simulink model "Model2"  (R2020a)
settings: Solver=VariableStepAuto  StartTime=0.0  StopTime=16*(1.302083333333333e-07)  RelTol=1e-3
undefined symbols (not defined in the file or in its folder): doppler, pskmod
libraries: commchan3 x2, commdigbbndpm3 x2, commutil2 x2, commrandsrc3 x1, commrflib2 x1, commsink2 x1
settings Model: Creator=esha_  LastModifiedBy=esha_

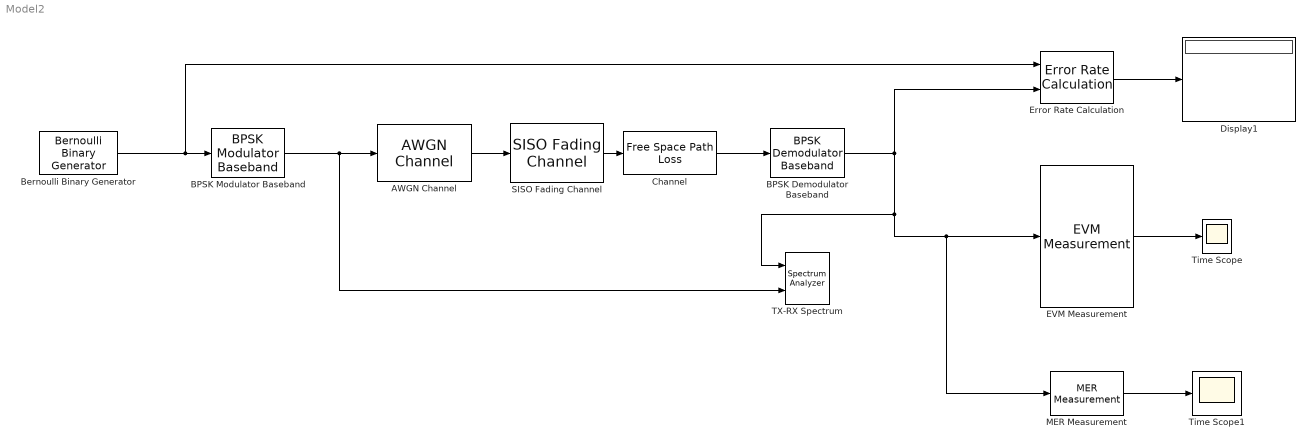
== system Model2 ==
  AWGN Channel : commchan3/AWGN Channel  InputProcessing=Columns as channels (frame based)  seed=67  noiseMode="Signal to noise ratio  (Eb/No)"  EbNodB=1  EsNodB=10  SNRdB=10  bitsPerSym=1  Ps=1  Tsym=0.000000065  variance=1
  BPSK Demodulator Baseband : commdigbbndpm3/BPSK Demodulator Baseband  DecType=Hard decision  VarSource=Dialog  Variance=1  Ph=0  outDtype=Inherit via internal rule  derotateFactorWordLen=16  derotateFactorDataTypeStr=Inherit: Same word length as input  derotateFactorLastDataTypeStr=Inherit: Same word length as input
  BPSK Modulator Baseband : commdigbbndpm3/BPSK Modulator Baseband  Ph=0  outDtype=double  outWordLen=16  outUDDataType=sfix(16)  outFracLenMode=Best precision  outFracLen=15  outDataTypeStr=double  outLastDataTypeStr=double
  Bernoulli Binary Generator : commrandsrc3/Bernoulli Binary Generator  ProbabilityOfZero=0.5  SeedSource=Parameter  Seed=61  SampleTime=1.302083333333333e-07  SamplesPerFrame=5000  OutputDataType=double  SimulateUsing=Code generation
  Channel : commrflib2/Free Space Path Loss  mode=Decibels  dB=50  d=0.100  fc=1920
      settings: SourceProductBaseCode=CM
  Display1 : Display
  EVM Measurement : commutil2/EVM Measurement  Normalization=Average reference signal power  AverageConstellationPower=1  PeakConstellationPower=1  ReferenceSignalSource=Estimated from reference constellation  ReferenceConstellation=pskmod((0:1),2,0)  MeasurementIntervalSource=Input length  MeasurementInterval=100  AveragingDimensions=1  MaximumEVMOutputPort=off  XPercentileEVMOutputPort=off  XPercentileValue=95  SymbolCountOutputPort=on  SimulateUsing=Interpreted execution
      settings: SourceProductBaseCode=CM
  Error Rate Calculation : commsink2/Error Rate Calculation  N=0  st_delay=0  cp_mode=Entire frame  subframe=[]  PMode=Port  WsName=ErrorVec  RsMode2=off  stop=on  numErr=100  maxBits=1e6
  MER Measurement : commutil2/MER Measurement  ReferenceSignalSource=Estimated from reference constellation  ReferenceConstellation=pskmod((0:1),2,0)  MeasurementIntervalSource=Input length  MeasurementInterval=100  AveragingDimensions=1  MinimumMEROutputPort=off  XPercentileMEROutputPort=off  XPercentileValue=95  SymbolCountOutputPort=off  SimulateUsing=Interpreted execution
      settings: SourceProductBaseCode=CM
  SISO Fading Channel : commchan3/SISO Fading Channel  InheritSampleRate=on  SampleRate=1  PathDelays=1.0e-06 *[0 0.2 0.4 0.8]  AveragePathGains="[0    -3    -6    -9]"  NormalizePathGains=on  FadingDistribution=Rayleigh  KFactor=3  DirectPathDopplerShift=0  DirectPathInitialPhase=0  MaximumDopplerShift=0.001  DopplerSpectrum=doppler('Jakes')  RandomStream=mt19937ar with seed  Seed=61  PathGainsOutputPort=off  ChannelFilterDelayOutputPort=off  SimulateUsing=Interpreted execution  Visualization=Frequency response  PathsForDopplerDisplay=1  SamplesToDisplay=100%
  TX-RX Spectrum : SpectrumAnalyzer  NumInputPorts=2
  Time Scope : Scope
      settings: Description=EVM
  Time Scope1 : Scope
      settings: Description=SNR
  wires:
  Bernoulli Binary Generator/1 -> Error Rate Calculation/1, BPSK Modulator Baseband/1
  Channel/1 -> BPSK Demodulator Baseband/1
  BPSK Demodulator Baseband/1 -> MER Measurement/1, EVM Measurement/1, TX-RX Spectrum/1, Error Rate Calculation/2
  EVM Measurement/1 -> Time Scope/1
  MER Measurement/1 -> Time Scope1/1
  Error Rate Calculation/1 -> Display1/1
  BPSK Modulator Baseband/1 -> TX-RX Spectrum/2, AWGN Channel/1
  AWGN Channel/1 -> SISO Fading Channel/1
  SISO Fading Channel/1 -> Channel/1
